simulink model "Chua_MPC"  (R2014a)
settings: Solver=ode4  StartTime=0.0  StopTime=T  FixedStep=Ts  RelTol=1e-8
values from neighbouring files (symbols this model uses):
  mpc = MPCController(model, N)    [Main_ChuaMPC.m]
  Ts = T/N    (= 0.01)    [Main_ChuaMPC.m]
  x0 = [0.02;0.05;-0.04;0.0002;0.0005;-0.0004]    [Main_ChuaMPC.m]
undefined symbols (not defined in the file or in its folder): MPCController
settings Model: Creator=gianni  LastModifiedBy=Gianni
settings DebuggingCC: MergeDetectMultiDrivingBlocksExec=error

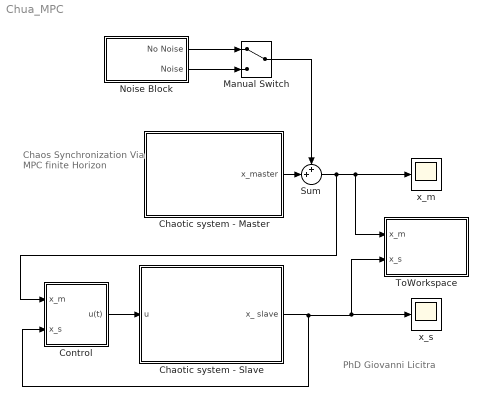
== system Chua_MPC ==
  note: PhD Giovanni Licitra
  note: Chaos Synchronization
      | Via MPC finite Horizon
  Chaotic system - Master : Subsystem
      mask Display: image('Chaos.jpg')
  Chaotic system - Slave : Subsystem
      mask Display: image('Chaos.jpg')
  Control : Subsystem
  Manual Switch : ManualSwitch
  Noise Block : Subsystem
  Sum : Sum  Inputs=++|
  ToWorkspace : Subsystem
  x_m : Scope
      settings: YMin=-1  YMax=0.5
  x_s : Scope
      settings: YMin=-1e+08  YMax=3e+08
  wires:
  Control/1(u(t)) -> Chaotic system - Slave/1(u)
  Sum/1 -> ToWorkspace/1(x_m), x_m/1, Control/1(x_m)
  Chaotic system - Slave/1(x_ slave) -> Control/2(x_s), ToWorkspace/2(x_s), x_s/1
  Chaotic system - Master/1(x_master) -> Sum/2
  Manual Switch/1 -> Sum/1
  Noise Block/1(No Noise) -> Manual Switch/1
  Noise Block/2(Noise) -> Manual Switch/2

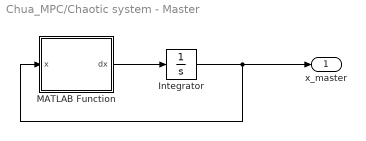
== system Chua_MPC/Chaotic system - Master ==
  Integrator : Integrator  InitialCondition=x0([1:3])
  MATLAB Function : MATLAB Function  TreatAsAtomicUnit=on
  x_master : Outport
  wires:
  Integrator/1 -> x_master/1, MATLAB Function/1(x)
  MATLAB Function/1(dx) -> Integrator/1

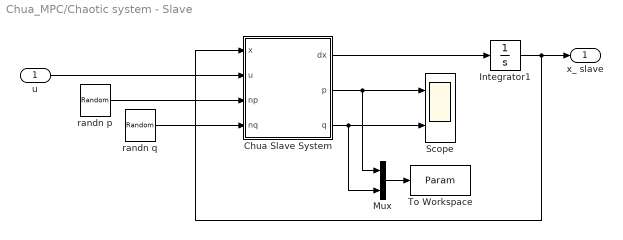
== system Chua_MPC/Chaotic system - Slave ==
  u : Inport
  Chua Slave System : MATLAB Function  TreatAsAtomicUnit=on
  Integrator1 : Integrator  InitialCondition=x0([4:6])
  Mux : Mux  Inputs=2
  Scope : Scope  NumInputPorts=2
      settings: YMin=9.5~13.6  YMax=10.5~14.8  SaveName=ScopeData4
  To Workspace : ToWorkspace  VariableName=Param  SaveFormat=Timeseries  SampleTime=-1
  randn p : UniformRandomNumber  Minimum=-0.5  Maximum=0.5  SampleTime=Ts
  randn q : UniformRandomNumber  Minimum=-0.5  Maximum=0.5  SampleTime=Ts
  x_ slave : Outport
  wires:
  Chua Slave System/1(dx) -> Integrator1/1
  Integrator1/1 -> Chua Slave System/1(x), x_ slave/1
  u/1 -> Chua Slave System/2(u)
  Chua Slave System/2(p) -> Mux/1, Scope/1
  Chua Slave System/3(q) -> Mux/2, Scope/2
  randn p/1 -> Chua Slave System/3(np)
  randn q/1 -> Chua Slave System/4(nq)
  Mux/1 -> To Workspace/1

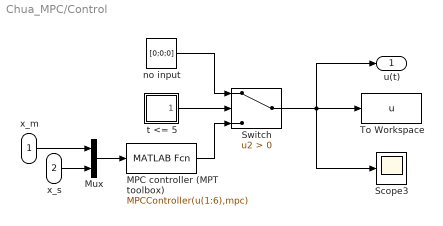
== system Chua_MPC/Control ==
  x_m : Inport
  x_s : Inport  Port=2
  MPC controller (MPT toolbox) : MATLABFcn  MATLABFcn=MPCController(u(1:6),mpc)
  Mux : Mux  Inputs=2
  Scope3 : Scope
      settings: YMin=-0.8  YMax=0.8  SaveName=ScopeData3
  Switch : Switch  Criteria=u2 > Threshold
  To Workspace : ToWorkspace  VariableName=u  SaveFormat=Timeseries  SampleTime=-1
  no input : Constant  Value=[0;0;0]
  t <= 5 : Subsystem
  u(t) : Outport
  wires:
  x_s/1 -> Mux/2
  x_m/1 -> Mux/1
  t <= 5/1(t <= 3) -> Switch/2
  no input/1 -> Switch/1
  Switch/1 -> Scope3/1, To Workspace/1, u(t)/1
  MPC controller (MPT toolbox)/1 -> Switch/3
  Mux/1 -> MPC controller (MPT toolbox)/1

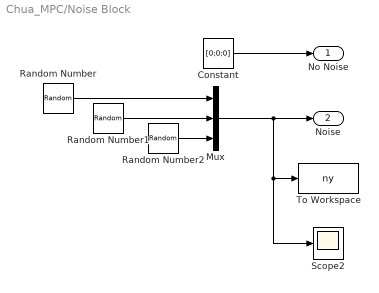
== system Chua_MPC/Noise Block ==
  Constant : Constant  Value=[0;0;0]
  Mux : Mux  Inputs=3
  Random Number : RandomNumber  Variance=0.001
  Random Number1 : RandomNumber  Variance=0.001
  Random Number2 : RandomNumber  Variance=0.001
  Scope2 : Scope
      settings: YMin=-0.6  YMax=0.6  SaveName=ScopeData6
  To Workspace : ToWorkspace  VariableName=ny  SaveFormat=Timeseries  SampleTime=-1
  No Noise : Outport
  Noise : Outport  Port=2
  wires:
  Random Number/1 -> Mux/1
  Random Number1/1 -> Mux/2
  Mux/1 -> Scope2/1, To Workspace/1, Noise/1
  Constant/1 -> No Noise/1
  Random Number2/1 -> Mux/3

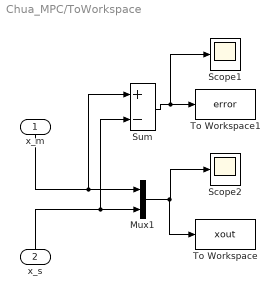
== system Chua_MPC/ToWorkspace ==
  x_m : Inport
  x_s : Inport  Port=2
  Mux1 : Mux  Inputs=2
  Scope1 : Scope
      settings: YMin=-0.5  YMax=0.4  SaveName=ScopeData5
  Scope2 : Scope
      settings: YMin=-0.6  YMax=0.6  SaveName=ScopeData2
  Sum : Sum  Inputs=+-
  To Workspace : ToWorkspace  VariableName=xout  SaveFormat=Timeseries  SampleTime=-1
  To Workspace1 : ToWorkspace  VariableName=error  SaveFormat=Timeseries  SampleTime=-1
  wires:
  Mux1/1 -> To Workspace/1, Scope2/1
  x_s/1 -> Sum/2, Mux1/2
  x_m/1 -> Sum/1, Mux1/1
  Sum/1 -> Scope1/1, To Workspace1/1

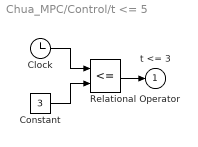
== system Chua_MPC/Control/t <= 5 ==
  Clock : Clock
  Constant : Constant  Value=3
  Relational Operator : RelationalOperator  Operator=<=  InputSameDT=on
  t <= 3 : Outport  InitialOutput=0
  wires:
  Constant/1 -> Relational Operator/2
  Clock/1 -> Relational Operator/1
  Relational Operator/1 -> t <= 3/1

== matlab function Chua_MPC/Chaotic system - Slave/Chua Slave System ==
  data: x input; dx output; u input; np input; nq input; p output; q output
function [dx,p,q] = ode(x,u,np,nq)                                   
    % INPUT:
    % np: additive uniform noise for p
    % nq: additive uniform noise for q
    % OUTPUT
    % p,q noisy
    
    % parameters with uncertainty
    p = 10+ np; 
    q = 100/7 + nq;                     
    x2 = x(1);y2 = x(2);z2 = x(3);    % slave states
    ux = u(1);uy = u(2); uz = u(3);   % control
    
    f_x1 = 2*x2^3 - x2/7;
    
    dx = [ p*(y2 - f_x1) + ux;
            x2 - y2 + z2 + uy;
          -q*y2 + uz;        
          ];  
end

== matlab function Chua_MPC/Chaotic system - Master/MATLAB Function ==
  data: x input; dx output
function dx = ode(x)                             
    p = 10;q = 100/7;                             % Parameters                 
    x1 = x(1);y1 = x(2);z1 = x(3);
    
    f_x1 = 2*x1^3 - x1/7;
    
    dx = [p*(y1-f_x1);
          x1-y1+z1;
          -q*y1;          
          ];  
end
